simulink model "modelS6"  (R2023b)
settings: Solver=ode45  StartTime=TSPAN(1)  StopTime=TSPAN(2)  MaxStep=MaxStep  RelTol=RelTol  AbsTol=AbsTol
undefined symbols (not defined in the file or in its folder): JSPAN, parameters, psi0, TSPAN, xi0
libraries: HyEQ_Library x1
settings Model: Creator=score  LastModifiedBy=zxz
settings DataIOCC: SaveFormat=Array  ReturnWorkspaceOutputs=off

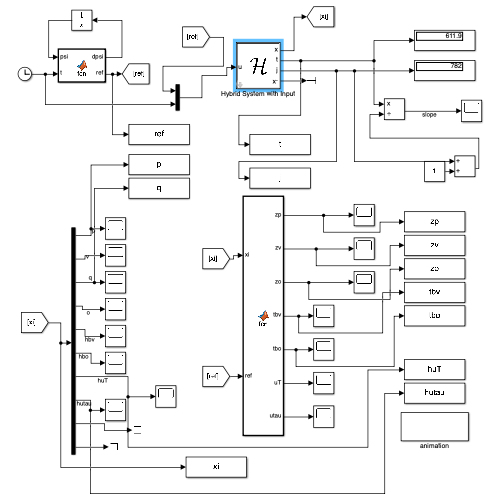
[thumbnail: Simulink's stored preview of the top-level diagram]
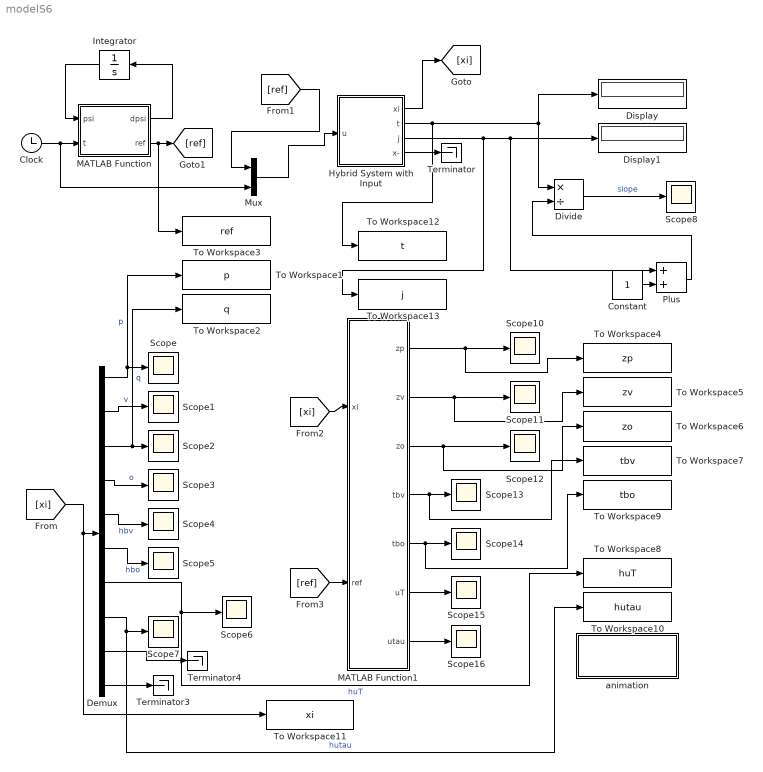
== system modelS6 ==
  Clock : Clock
  Constant : Constant
  Demux : Demux  Outputs=[2;2;2;1;2;1;1;1;1;1]
  Display : Display
  Display1 : Display
  Divide : Product  Inputs=*/
  Hybrid System with Input : Subsystem  LoadFcn=set_param(gcb,'LinkStatus','none')  mask(Hybrid System with Inputs){x0=xi0, input_dim=9, parameters=parameters, T=TSPAN(2), J=JSPAN(2), rule=Flow}
      mask prompts: x0 "Initial Condition (column vector)"; input_dim "Input Dimension (positive integer)"; T "Flow Horizon (nonnegative real)"; J "Jump Horizon (nonnegative integer)"; rule "Flow/Jump Priorty Rule"
      mask help:
      | To modify (f, g, C, D) for this block, "Look inside" the block mask by either clicking the down arrow in the lower-left corner or selecting "Mask" > "Look Under Mask" from the context menu.
      |
      | For instructions how to use this block, see the
      mask init:
      | state_dim = numel(x0);
      settings: CopyFcn=|
      | set_param(gcb,'LinkStatus','none'),
      | set_param(gcs, 'MaxStep', 'MaxStep', 'RelTol', 'RelTol','StopTime', 'T')
      mask Help:
      | To modify (f, g, C, D) for this block, "Look inside" the block mask by either clicking the down arrow in the lower-left corner or selecting "Mask" > "Look Under Mask" from the context menu.
      | 
      | The value given in the 'parameters' field is passed as the last input argument for f, g, C, and D. Any MATLAB object can be used, but we recommend using a struct. For example, in the initialization script, a parameters struct can be defined as followed.
      |   parameters = struct();
      |   parameters.A = eye(2);
      |   parameters.B = [1; 0];
      | 
      | The output "x-" is the state output delayed by one integration step. Use this output to break algebraic loops.
      mask TypeOptions x0: Integrator System/x0
      mask TypeOptions T: Integrator System/T
      mask TypeOptions J: Integrator System/J
      mask TypeOptions rule: Jump | Flow | Random
      mask DialogControl Control2 Prompt: Introduction to the HyEQ Simulink-based Library
      mask DialogControl Control2 Callback: hybrid.internal.openHelp('Help_SimulinkLibrary')
      mask DialogControl Container3 Prompt: System Configuration
      mask DialogControl Container2 Prompt: Solver Options
      mask Display:
      | image('Hcal.jpg')
      | port_label('output', 1, 'x')
      | port_label('output', 2, 't')
      | port_label('output', 3, 'j')
      | port_label('output', 4, 'x^-','texmode', 'on')
      | port_label('input', 1, 'u')
  Integrator : Integrator  InitialCondition=psi0
  MATLAB Function : MATLAB Function  TreatAsAtomicUnit=on
  MATLAB Function1 : MATLAB Function  TreatAsAtomicUnit=on
  Mux : Mux  Inputs=2
  Plus : Sum
  Scope{,1..8,10..16} (16 alike) : Scope
  Terminator : Terminator
  Terminator3 : Terminator
  Terminator4 : Terminator
  To Workspace1 : ToWorkspace  VariableName=p  SampleTime=-1
  To Workspace10 : ToWorkspace  VariableName=hutau  SampleTime=-1
  To Workspace11 : ToWorkspace  VariableName=xi  SampleTime=-1
  To Workspace12 : ToWorkspace  VariableName=t  SampleTime=-1
  To Workspace13 : ToWorkspace  VariableName=j  SampleTime=-1
  To Workspace2 : ToWorkspace  VariableName=q  SampleTime=-1
  To Workspace3 : ToWorkspace  VariableName=ref  SampleTime=-1
  To Workspace4 : ToWorkspace  VariableName=zp  SampleTime=-1
      settings: Save2DSignal=2-D array (concatenate along first dimension)
  To Workspace5 : ToWorkspace  VariableName=zv  SampleTime=-1
  To Workspace6 : ToWorkspace  VariableName=zo  SampleTime=-1
  To Workspace7 : ToWorkspace  VariableName=tbv  SampleTime=-1
  To Workspace8 : ToWorkspace  VariableName=huT  SampleTime=-1
  To Workspace9 : ToWorkspace  VariableName=tbo  SampleTime=-1
  animation : Subsystem
      settings: OpenFcn=|
      | pd0=ref(:,1:2);
      | %%%%animation
      | figure(100);
      | Speedy=0.5/MaxStep;
      | for i=1:Speedy:length(tout)
      |     %past locations
      |     plot(pd0(1:i,1),pd0(1:i,2),'ro','MarkerSize',2);hold on;
      |     plot(p(1:i,1),p(1:i,2),'bo','MarkerSize',1);hold on;
      |     %current location
      |     plot(pd0(i,1),pd0(i,2),'ro','MarkerSize',14);hold on;
      |     plot(p(i,1),p(i,2),'bo','MarkerSize',7);hold on;
      |     %initial location
      |     plot(pd0(1,1),pd0(1,2),'rx','MarkerSize',14);hold on;
      |     plot(p(1,1),p(1,2),'bx','MarkerSize',7);hold on;
      |     %current xB axis (e1) to be expressed in I
      |     R=q2rot(q(i,:));
      |     xB_I=10.*R*[1;0];
      |     arrow_ini=p(i,1:2)';
      |     arrow_end=arrow_ini + xB_I;
      |     plot(linspace(arrow_ini(1),arrow_end(1),10),linspace(arrow_ini(2),arrow_end(2),10),'LineWidth',2);hold on;
      |     %force disturbance bv
      |     arrow_ini=[0;0];
      |     arrow_end=arrow_ini + 10.*bv./norm(bv);
      |     plot(linspace(arrow_ini(1),arrow_end(1),10),linspace(arrow_ini(2),arrow_end(2),10),'LineWidth',2);hold on;
      |     %torque disturbance bo
      |     plot(p(i,1),p(i,2),'bx','MarkerSize',3); hold off;
      |     insidePaper=-abs(bo);
      |     text(p(i,1)+5,p(i,2)+5,num2str(insidePaper));
      |     grid on;axis equal;
      |     xlabel('x');ylabel('y');
      |     axis([-50 50 -50 50]);
      |     timer=tout(i);
      |     text(49,49,num2str(timer));
      |     %set(gca,'Ydir','reverse')
      |     pause(0.001)
      |     % pause(0.1)
      | end
  wires:
  Hybrid System with Input/4(x-) -> Terminator/1
  Clock/1 -> Mux/2, MATLAB Function/2(t)
  MATLAB Function/1(dpsi) -> Integrator/1
  Integrator/1 -> MATLAB Function/1(psi)
  Hybrid System with Input/2(t) -> To Workspace12/1, Divide/1, Display/1
  Hybrid System with Input/3(j) -> To Workspace13/1, Plus/1, Display1/1
  Hybrid System with Input/1(xi) -> [xi]
  [xi] -> To Workspace11/1, Demux/1
  Demux/1 -> To Workspace1/1, Scope/1  "p"
  Demux/2 -> Scope1/1  "v"
  Demux/3 -> To Workspace2/1, Scope2/1  "q"
  Demux/4 -> Scope3/1  "o"
  Demux/5 -> Scope4/1  "hbv"
  Demux/6 -> Scope5/1  "hbo"
  Demux/7 -> Scope6/1, To Workspace8/1  "huT"
  Demux/8 -> Scope7/1, To Workspace10/1  "hutau"
  MATLAB Function1/7(utau) -> Scope16/1
  MATLAB Function1/4(tbv) -> To Workspace7/1, Scope13/1
  MATLAB Function1/6(uT) -> Scope15/1
  MATLAB Function1/5(tbo) -> To Workspace9/1, Scope14/1
  MATLAB Function1/1(zp) -> To Workspace4/1, Scope10/1
  MATLAB Function1/2(zv) -> To Workspace5/1, Scope11/1
  MATLAB Function1/3(zo) -> To Workspace6/1, Scope12/1
  [xi] -> MATLAB Function1/1(xi)
  MATLAB Function/2(ref) -> To Workspace3/1, [ref]
  [ref] -> MATLAB Function1/2(ref)
  Constant/1 -> Plus/2
  Plus/1 -> Divide/2
  Divide/1 -> Scope8/1  "slope"
  Demux/10 -> Terminator3/1
  Demux/9 -> Terminator4/1
  [ref] -> Mux/1
  Mux/1 -> Hybrid System with Input/1(u)

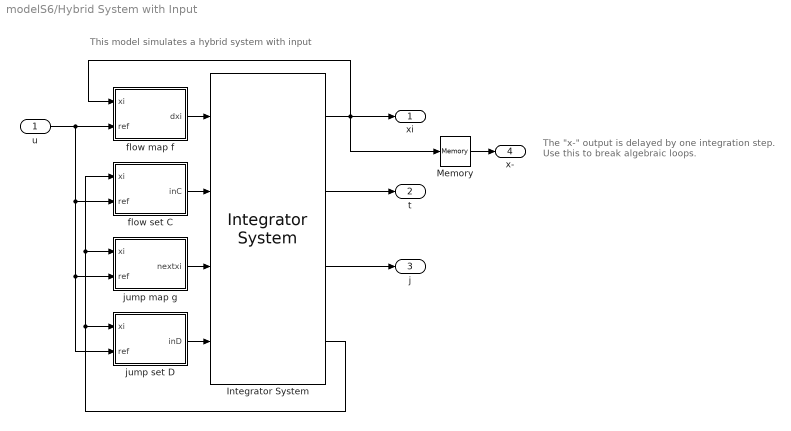
== system modelS6/Hybrid System with Input ==
  note: This model simulates a hybrid system with input
  note: The "x-" output is delayed by one integration step. Use this to break algebraic loops.
  u : Inport  PortDimensions=input_dim
  Integrator System : HyEQ_Library/Other/Integrator System  Priority=2  T=T  J=J  x0=x0  rule=rule
      settings: SourceProductName=Hybrid Equations Toolbox
  Memory : Memory  InitialCondition=x0
  flow map f : MATLAB Function  TreatAsAtomicUnit=on
  flow set C : MATLAB Function  TreatAsAtomicUnit=on
  jump map g : MATLAB Function  TreatAsAtomicUnit=on
  jump set D : MATLAB Function  TreatAsAtomicUnit=on
  xi : Outport  PortDimensions=state_dim
  t : Outport  Port=2  PortDimensions=1
  j : Outport  Port=3  PortDimensions=1
  x- : Outport  Port=4  PortDimensions=state_dim
  wires:
  Memory/1 -> x-/1
  jump map g/1(nextxi) -> Integrator System/3
  jump set D/1(inD) -> Integrator System/4
  u/1 -> jump set D/2(ref), jump map g/2(ref), flow set C/2(ref), flow map f/2(ref)
  Integrator System/3 -> j/1
  Integrator System/2 -> t/1
  flow set C/1(inC) -> Integrator System/2
  Integrator System/1 -> xi/1, flow map f/1(xi), Memory/1
  Integrator System/4 -> jump map g/1(xi), flow set C/1(xi), jump set D/1(xi)
  flow map f/1(dxi) -> Integrator System/1

== system modelS6/animation ==

== matlab function modelS6/MATLAB Function1 ==
  data: xi input; zp output; ref input; zv output; zo output; tbv output; tbo output; parameters parameter; uT output; utau output
function [zp,zv,zo,tbv,tbo, uT,utau] = fcn(xi,ref,parameters)

e1=parameters.e1;
e2=parameters.e2;
S=parameters.S;
M=parameters.M;
J=parameters.J;
D_l=parameters.D_l;
d_o=parameters.d_o;
d_q=parameters.d_q;

bv=parameters.bv;
bo=parameters.bo;

delta=parameters.delta;
kp=parameters.kp;
kv=parameters.kv;
ko=parameters.ko;
% hp=parameters.hp;
hv=parameters.hv;
ho=parameters.ho;

pd0=ref(1:2);
pd1=ref(3:4);
pd2=ref(5:6);
pd3=ref(7:8);

p=xi(1:2);
v=xi(3:4);
q=xi(5:6);
o=xi(7);
hbv=xi(8:9);
hbo=xi(10);


invM=inv(M);
invJ=inv(J);

R=q2rot(q);
zp=p-pd0;
s=sigma(zp,parameters);
Ds=Dsigma(zp,parameters);
% DDs=DDsigma(zp,parameters);

fp=R*v-pd1;
zv=v - R'*pd1 + kp.*invM*R'*s - delta;

phi=(M*S-S*M)*R'*pd1 - S*M*delta;
eta=inv(hv).*invM*R'*s + kp.*R'*Ds*fp...
    + kv.*inv(hv).*invM*zv - M*R'*pd2 - D_l*v...
    - d_q.*(e1'*v)*abs(e1'*v).*e1 + R'*hbv;


%====================================================================

zo=e2'*(phi*o + eta);

tbv=hbv-bv;
tbo=hbo-bo;

%====================================================================
uT=kappaT(xi,ref,parameters);
utau=kappatau(xi,ref,parameters);

== matlab function modelS6/MATLAB Function ==
  data: psi input; dpsi output; t input; ref output; parameters parameter
function [dpsi,ref] = fcn(psi,t,parameters)
c_max=parameters.c_max;
o1=parameters.o1;
psi1=parameters.psi1;
o2=parameters.o2;
psi2=parameters.psi2;
v_max=parameters.v_max;

% % % normal curve
% pd0=c_max.*[sin(o1*t+psi1);sin(o2*t+psi2)];
% pd1=c_max.*[o1*cos(o1*t+psi1);o2*cos(o2*t+psi2)];
% pd2=-diag([o1^2;o2^2])*pd0;
% pd3=-diag([o1^2;o2^2])*pd1;
% dpsi=0;%auxiliary

%Lissajous Curve
Dphi_=Dphi(psi,parameters);
DDphi_=DDphi(psi,parameters);
DDDphi_=DDDphi(psi,parameters);

dpsi=v_max*inv(norm(Dphi_));
ddpsi=-v_max.*(norm(Dphi_))^(-3).*Dphi_'*DDphi_*dpsi;

f=Drho(Dphi_);
g=DDphi_*dpsi;
h=DDphi_;
Df=DDrho(Dphi_)*DDphi_*dpsi;
Dh=DDDphi_*dpsi;
Dg=kron(dpsi,eye(2))*Dh + h*ddpsi;

pd0=c_max.*[sin(o1*psi+psi1);sin(o2*psi+psi2)];
pd1=v_max.*rho(Dphi_);
pd2=v_max.*Drho(Dphi_)*DDphi_*dpsi;
pd3=v_max.*( kron(g',eye(2))*Df + f*Dg );

ref=[pd0;pd1;pd2;pd3];

end

function out=Dphi(theta,parameters)
    c_max=parameters.c_max;
    o1=parameters.o1;
    psi1=parameters.psi1;
    o2=parameters.o2;
    psi2=parameters.psi2;
    out=c_max.*[o1*cos(o1*theta+psi1);o2*cos(o2*theta+psi2)];
end

function out=DDphi(theta,parameters)
    c_max=parameters.c_max;
    o1=parameters.o1;
    psi1=parameters.psi1;
    o2=parameters.o2;
    psi2=parameters.psi2;
    out=c_max.*[-o1*o1*sin(o1*theta+psi1);-o2*o2*sin(o2*theta+psi2)];
end

function out=DDDphi(theta,parameters)
    c_max=parameters.c_max;
    o1=parameters.o1;
    psi1=parameters.psi1;
    o2=parameters.o2;
    psi2=parameters.psi2;
    out=c_max.*[-o1*o1*o1*cos(o1*theta+psi1);-o2*o2*o2*cos(o2*theta+psi2)];
end

function out=rho(x)
    out=x./norm(x);
end

function out=Drho(x)
    out=inv(norm(x)).*(eye(2)-rho(x)*rho(x)');
end

function out=DDrho(x)
    rho_=rho(x);
    Drho_=Drho(x);
    out=-inv(norm(x)).*( reshape(Drho_,[4,1])*rho_' + ( kron(rho_,eye(2)) + kron(eye(2),rho_) )*Drho_ );
end

== matlab function modelS6/Hybrid System with Input/flow map f ==
  data: xi input size=state_dim; ref input size=input_dim; dxi output size=state_dim; parameters parameter
function dxi = f(xi, ref, parameters)

timer=ref(end);
ref=ref(1:end-1);
e1=parameters.e1;
S=parameters.S;
M=parameters.M;
D_l=parameters.D_l;
d_o=parameters.d_o;
d_q=parameters.d_q;
J=parameters.J;
bv=parameters.bv;
bo=parameters.bo;

p=xi(1:2);
v=xi(3:4);
q=xi(5:6);
o=xi(7);
% hbv=xi(8:9);
% hbo=xi(10);
huT=xi(11);
hutau=xi(12);
timer=xi(13);
Vcal=xi(14);

% [dpsi,ref_] = ref(psi,timer,parameters);


invM=inv(M);
invJ=inv(J);
R=q2rot(q);

bv_1=bv(1);
bv_2=bv(2);
bo_=bo;
bv=[bv_1*sin(0.1*timer);bv_2*sin(0.2*timer)];
bo=bo_*cos(0.15*timer);

% uT=kappaT(xi,ref,parameters);
% utau=kappatau(xi,ref,parameters);

dp=R*v;
dv=-invM*S*M*v*o - invM*D_l*v - d_q.*(e1'*v)*abs(e1'*v).*invM*e1 + invM*R'*bv + huT.*invM*e1;
dq=0.5.*S*q*o;
do=-invJ*d_o*o + invJ*bo + invJ*hutau;

dhbv=chiv(xi,ref,parameters);%have access to the real plant state
dhbo=chio(xi,ref,parameters);%have access to the real plant state

dhuT=0;
dhutau=0;
dtimer=1;
dVcal_=dVcal(xi,ref,parameters);

dxi=[dp;dv;dq;do;dhbv;dhbo; dhuT;dhutau; dtimer;dVcal_];
end

== matlab function modelS6/Hybrid System with Input/flow set C ==
  data: xi input size=state_dim; ref input size=input_dim; inC output size=1; parameters parameter
function inC = C(xi, ref, parameters)
timer=ref(end);
ref=ref(1:end-1);
uSlopeThreshold=parameters.uSlopeThreshold;

huT=xi(11);
hutau=xi(12);

next_huT=kappaT(xi,ref,parameters);
next_hutau=kappatau(xi,ref,parameters);

u_err=norm([huT-next_huT;hutau-next_hutau]);

if u_err<=uSlopeThreshold*norm([huT;hutau])
   inC=1;
else
    inC=0;
end
end

== matlab function modelS6/Hybrid System with Input/jump map g ==
  data: xi input size=state_dim; ref input size=input_dim; nextxi output size=state_dim; parameters parameter
function nextxi = g(xi, ref, parameters)
timer=ref(end);
ref=ref(1:end-1);
p=xi(1:2);
v=xi(3:4);
q=xi(5:6);
o=xi(7);
hbv=xi(8:9);
hbo=xi(10);
% huT=xi(11);
% hutau=xi(12);
timer=xi(13);
Vcal=xi(14);

next_huT=kappaT(xi,ref,parameters);
next_hutau=kappatau(xi,ref,parameters);
next_timer=0;

nextxi=[p;v;q;o;hbv;hbo; next_huT;next_hutau; next_timer;Vcal];
end

== matlab function modelS6/Hybrid System with Input/jump set D ==
  data: xi input size=state_dim; ref input size=input_dim; inD output size=1; parameters parameter
function inD = D(xi, ref, parameters)
timer=ref(end);
ref=ref(1:end-1);
uSlopeThreshold=parameters.uSlopeThreshold;

huT=xi(11);
hutau=xi(12);

next_huT=kappaT(xi,ref,parameters);
next_hutau=kappatau(xi,ref,parameters);

u_err=norm([huT-next_huT;hutau-next_hutau]);

if u_err>=uSlopeThreshold*norm([huT;hutau])
   inD=1;
else
    inD=0;
end
end
